simulink model "NHR9410Model96k_2020b"  (R2020b)
settings: Solver=ode45  StartTime=0.0  StopTime=1  FixedStep=0.001  MaxStep=20e-6  RelTol=1e-3
undefined symbols (not defined in the file): Ts
libraries: simulink x85, fl_lib x49, powerlib_meascontrol x27, simulink_extras x24, nesl_utility x13
(part 2 of 4)

== system NHR9410Model96k_2020b/NHR 9410/Chanel-3 ==
  satefy_trip : Inport
  HW Mode Selection : Inport  Port=2
  Ch-3 input [P V I] : Inport  Port=3
  Chanel-3 Control : Subsystem
  Constant : Constant  Value=p_switch
  Constant4 : Constant  Value=0.1
  Current Sensor : fl_lib/Electrical/Electrical Sensors/Current Sensor
  Logical Operator : Logic  AllPortsSameDT=off  OutDataTypeStr=boolean
  Logical Operator1 : Logic  Operator=NOT  AllPortsSameDT=off  OutDataTypeStr=boolean
  NHR 9410 : fl_lib/Electrical/Electrical Sources/Controlled Voltage Source
  PS Constant : fl_lib/Physical Signals/Sources/PS Constant  constant=0
  PS Product1 : fl_lib/Physical Signals/Functions/PS Product
  PS-Simulink Converter1 : nesl_utility/PS-Simulink Converter  PhysicalDomain=network_engine_domain  SubClassName=ps_output  LeftPortType=input  RightPortType=output  PseudoPeriodic=off  Frequencies=[]  Unit=inherit  AffineConversion=off
  PS-Simulink Converter2 : nesl_utility/PS-Simulink Converter  PhysicalDomain=network_engine_domain  SubClassName=ps_output  LeftPortType=input  RightPortType=output  PseudoPeriodic=off  Frequencies=[]  Unit=1  AffineConversion=off
  PS-Simulink Converter4 : nesl_utility/PS-Simulink Converter  PhysicalDomain=network_engine_domain  SubClassName=ps_output  LeftPortType=input  RightPortType=output  PseudoPeriodic=off  Frequencies=[]  Unit=1  AffineConversion=off
  Series Resistor : fl_lib/Electrical/Electrical Elements/Variable Resistor  Rmin=0.0001 Ohm  i_specify=off  i_priority=None  i=0 A  i_nominal_specify=off  i_nominal_unit=A  i_nominal_value=1  v_specify=off  v_priority=None  v=0 V  v_nominal_specify=off  v_nominal_unit=V  v_nominal_value=1
  Simulink-PS Converter : nesl_utility/Simulink-PS Converter  PhysicalDomain=network_engine_domain  SubClassName=ps_input  LeftPortType=input  RightPortType=output  PseudoPeriodic=off  Frequencies=[]  NoiseDistribution=none  NoiseParameters=[]  Unit=1  AffineConversion=off  FilteringAndDerivatives=filter  SimscapeFilterOrder=1  InputFilterTimeConstant=0.001  UdotUserProvided=0
  Switch : Switch  Criteria=u2 > Threshold  ZeroCross=off
  Voltage Sensor1 : fl_lib/Electrical/Electrical Sensors/Voltage Sensor
  + : PMIOPort  Tag=PMCPort  Side=Left
  - : PMIOPort  Tag=PMCPort  Port=2  Side=Left
  Pout : Outport  VectorParamsAs1DForOutWhenUnconnected=off
  Vout : Outport  Port=2  VectorParamsAs1DForOutWhenUnconnected=off
  Iout : Outport  Port=3  VectorParamsAs1DForOutWhenUnconnected=off
  wires:
  PS-Simulink Converter2/1 -> Iout/1, Chanel-3 Control/3(Iout)
  PS-Simulink Converter4/1 -> Vout/1, Chanel-3 Control/2(Vout)
  PS-Simulink Converter1/1 -> Pout/1, Chanel-3 Control/1(Pout)
  HW Mode Selection/1 -> Chanel-3 Control/5(HW mode selection)
  Ch-3 input [P V I]/1 -> Chanel-3 Control/4(Ch-3 input [P V I])
  Constant4/1 -> Switch/3
  Chanel-3 Control/1(Vin) -> Switch/1
  Switch/1 -> Simulink-PS Converter/1
  Logical Operator1/1 -> Logical Operator/2
  satefy_trip/1 -> Logical Operator1/1
  Constant/1 -> Logical Operator/1
  Logical Operator/1 -> Switch/2
  connections:
  Current Sensor/LConn1 -- Series Resistor/RConn1
  PS Constant/RConn1 -- Series Resistor/LConn1
  PS Product1/RConn1 -- PS-Simulink Converter1/LConn1
  Series Resistor/LConn2 -- NHR 9410/LConn1
  Simulink-PS Converter/RConn1 -- NHR 9410/RConn1
  Voltage Sensor1/LConn1 -- +/RConn1 -- Current Sensor/RConn2
  PS-Simulink Converter2/LConn1 -- PS Product1/LConn1 -- Current Sensor/RConn1
  NHR 9410/RConn2 -- -/RConn1 -- Voltage Sensor1/RConn2
  Voltage Sensor1/RConn1 -- PS Product1/LConn2 -- PS-Simulink Converter4/LConn1

== system NHR9410Model96k_2020b/NHR 9410 Safety Settings/Safety Ch-1 ==
  ch-1 out : Inport
  peak_ctrl : Inport  Port=2
  Demux : Demux  Outputs=8
  Logical Operator : Logic  Operator=OR  Inputs=8  AllPortsSameDT=off  OutDataTypeStr=boolean
  Mux : Mux  Inputs=9
  Trip signal generator (max) Sink Current : Subsystem  mask{trip_thres=Imaxsnk1, trip_t=Timaxsnk1}
      mask prompts: trip_thres "Tripping Threshold (max)"; trip_t "Trip Time"
  Trip signal generator (max) Sink Power : Subsystem  mask{trip_thres=Pmaxsnk1, trip_t=Tpmaxsnk1}
      mask prompts: trip_thres "Tripping Threshold (max)"; trip_t "Trip Time"
  Trip signal generator (max) Source Current : Subsystem  mask{trip_thres=Imaxsrc1, trip_t=Timaxsrc1}
      mask prompts: trip_thres "Tripping Threshold (max)"; trip_t "Trip Time"
  Trip signal generator (max) Source Power : Subsystem  mask{trip_thres=Pmaxsrc1, trip_t=Tpmaxsrc1}
      mask prompts: trip_thres "Tripping Threshold (max)"; trip_t "Trip Time"
  Trip signal generator (max) Voltage : Subsystem  mask{trip_thres=Vmax1, trip_t=Tvmax1}
      mask prompts: trip_thres "Tripping Threshold (max)"; trip_t "Trip Time"
  Trip signal generator (min) Voltage : Subsystem  mask{trip_thres=Vmin1, trip_t=Tvmin1}
      mask prompts: trip_thres "Tripping Threshold (max)"; trip_t "Trip Time"
  Trip signal generator (peak) Current : Subsystem  mask{trip_thres=Ipeak1}
      mask prompts: trip_thres "Tripping Threshold (max)"
  Trip signal generator (peak) Voltage : Subsystem  mask{trip_thres=Vpeak1}
      mask prompts: trip_thres "Tripping Threshold (max)"
  ch-1 trip : Outport  VectorParamsAs1DForOutWhenUnconnected=off
  ch-1 trip_all : Outport  Port=2  VectorParamsAs1DForOutWhenUnconnected=off
  wires:
  Demux/1 -> Trip signal generator (min) Voltage/1(signal_in)
  Demux/2 -> Trip signal generator (max) Voltage/1(signal_in)
  Demux/5 -> Trip signal generator (max) Sink Current/1(signal_in)
  Trip signal generator (max) Sink Current/1(signal_trip) -> Mux/6, Logical Operator/5
  Demux/4 -> Trip signal generator (max) Source Current/1(signal_in)
  ch-1 out/1 -> Demux/1
  Trip signal generator (min) Voltage/1(signal_trip) -> Mux/2, Logical Operator/1
  Trip signal generator (max) Source Current/1(signal_trip) -> Mux/5, Logical Operator/4
  Trip signal generator (peak) Voltage/1(signal_trip) -> Mux/4, Logical Operator/3
  Trip signal generator (peak) Current/1(signal_trip) -> Mux/7, Logical Operator/6
  Demux/8 -> Trip signal generator (max) Sink Power/1(signal_in)
  Trip signal generator (max) Voltage/1(signal_trip) -> Mux/3, Logical Operator/2
  Trip signal generator (max) Sink Power/1(signal_trip) -> Mux/9, Logical Operator/8
  Demux/3 -> Trip signal generator (peak) Voltage/1(signal_in)
  Trip signal generator (max) Source Power/1(signal_trip) -> Mux/8, Logical Operator/7
  Demux/7 -> Trip signal generator (max) Source Power/1(signal_in)
  Demux/6 -> Trip signal generator (peak) Current/1(signal_in)
  Logical Operator/1 -> Mux/1, ch-1 trip/1
  peak_ctrl/1 -> Trip signal generator (peak) Voltage/2(peak_ctrl), Trip signal generator (peak) Current/2(peak_ctrl)
  Mux/1 -> ch-1 trip_all/1

== system NHR9410Model96k_2020b/NHR 9410 Safety Settings/Safety Ch-2 ==
  ch-2 out : Inport
  peak_ctrl : Inport  Port=2
  Demux : Demux  Outputs=8
  Logical Operator : Logic  Operator=OR  Inputs=8  AllPortsSameDT=off  OutDataTypeStr=boolean
  Mux : Mux  Inputs=9
  Trip signal generator (max) Sink Current : Subsystem  mask{trip_thres=Imaxsnk2, trip_t=Timaxsnk2}
      mask prompts: trip_thres "Tripping Threshold (max)"; trip_t "Trip Time"
  Trip signal generator (max) Sink Power : Subsystem  mask{trip_thres=Pmaxsnk2, trip_t=Tpmaxsnk2}
      mask prompts: trip_thres "Tripping Threshold (max)"; trip_t "Trip Time"
  Trip signal generator (max) Source Current : Subsystem  mask{trip_thres=Imaxsrc2, trip_t=Timaxsrc2}
      mask prompts: trip_thres "Tripping Threshold (max)"; trip_t "Trip Time"
  Trip signal generator (max) Source Power : Subsystem  mask{trip_thres=Pmaxsrc2, trip_t=Tpmaxsrc2}
      mask prompts: trip_thres "Tripping Threshold (max)"; trip_t "Trip Time"
  Trip signal generator (max) Voltage : Subsystem  mask{trip_thres=Vmax2, trip_t=Tvmax2}
      mask prompts: trip_thres "Tripping Threshold (max)"; trip_t "Trip Time"
  Trip signal generator (min) Voltage : Subsystem  mask{trip_thres=Vmin2, trip_t=Tvmin2}
      mask prompts: trip_thres "Tripping Threshold (max)"; trip_t "Trip Time"
  Trip signal generator (peak) Current : Subsystem  mask{trip_thres=Ipeak2}
      mask prompts: trip_thres "Tripping Threshold (max)"
  Trip signal generator (peak) Voltage : Subsystem  mask{trip_thres=Vpeak2}
      mask prompts: trip_thres "Tripping Threshold (max)"
  ch-2 trip : Outport  VectorParamsAs1DForOutWhenUnconnected=off
  ch-2 trip_all : Outport  Port=2  VectorParamsAs1DForOutWhenUnconnected=off
  wires:
  Logical Operator/1 -> Mux/1, ch-2 trip/1
  Demux/6 -> Trip signal generator (peak) Current/1(signal_in)
  Demux/7 -> Trip signal generator (max) Source Power/1(signal_in)
  Trip signal generator (max) Source Power/1(signal_trip) -> Mux/8, Logical Operator/7
  Demux/3 -> Trip signal generator (peak) Voltage/1(signal_in)
  Trip signal generator (max) Sink Power/1(signal_trip) -> Mux/9, Logical Operator/8
  Trip signal generator (max) Voltage/1(signal_trip) -> Mux/3, Logical Operator/2
  Demux/8 -> Trip signal generator (max) Sink Power/1(signal_in)
  Trip signal generator (peak) Current/1(signal_trip) -> Mux/7, Logical Operator/6
  Trip signal generator (peak) Voltage/1(signal_trip) -> Mux/4, Logical Operator/3
  Trip signal generator (max) Source Current/1(signal_trip) -> Mux/5, Logical Operator/4
  Trip signal generator (min) Voltage/1(signal_trip) -> Mux/2, Logical Operator/1
  ch-2 out/1 -> Demux/1
  Demux/4 -> Trip signal generator (max) Source Current/1(signal_in)
  Demux/5 -> Trip signal generator (max) Sink Current/1(signal_in)
  Demux/2 -> Trip signal generator (max) Voltage/1(signal_in)
  Demux/1 -> Trip signal generator (min) Voltage/1(signal_in)
  peak_ctrl/1 -> Trip signal generator (peak) Voltage/2(peak_ctrl), Trip signal generator (peak) Current/2(peak_ctrl)
  Mux/1 -> ch-2 trip_all/1
  Trip signal generator (max) Sink Current/1(signal_trip) -> Mux/6, Logical Operator/5

== system NHR9410Model96k_2020b/NHR 9410 Safety Settings/Safety Ch-3 ==
  ch-3 out : Inport
  peak_ctrl : Inport  Port=2
  Demux : Demux  Outputs=8
  Logical Operator : Logic  Operator=OR  Inputs=8  AllPortsSameDT=off  OutDataTypeStr=boolean
  Mux : Mux  Inputs=9
  Trip signal generator (max) Sink Current : Subsystem  mask{trip_thres=Imaxsnk3, trip_t=Timaxsnk3}
      mask prompts: trip_thres "Tripping Threshold (max)"; trip_t "Trip Time"
  Trip signal generator (max) Sink Power : Subsystem  mask{trip_thres=Pmaxsnk3, trip_t=Tpmaxsnk3}
      mask prompts: trip_thres "Tripping Threshold (max)"; trip_t "Trip Time"
  Trip signal generator (max) Source Current : Subsystem  mask{trip_thres=Imaxsrc3, trip_t=Timaxsrc3}
      mask prompts: trip_thres "Tripping Threshold (max)"; trip_t "Trip Time"
  Trip signal generator (max) Source Power : Subsystem  mask{trip_thres=Pmaxsrc3, trip_t=Tpmaxsrc3}
      mask prompts: trip_thres "Tripping Threshold (max)"; trip_t "Trip Time"
  Trip signal generator (max) Voltage : Subsystem  mask{trip_thres=Vmax3, trip_t=Tvmax3}
      mask prompts: trip_thres "Tripping Threshold (max)"; trip_t "Trip Time"
  Trip signal generator (min) Voltage : Subsystem  mask{trip_thres=Vmin3, trip_t=Tvmin3}
      mask prompts: trip_thres "Tripping Threshold (max)"; trip_t "Trip Time"
  Trip signal generator (peak) Current : Subsystem  mask{trip_thres=Ipeak3}
      mask prompts: trip_thres "Tripping Threshold (max)"
  Trip signal generator (peak) Voltage : Subsystem  mask{trip_thres=Vpeak3}
      mask prompts: trip_thres "Tripping Threshold (max)"
  ch-3 trip : Outport  VectorParamsAs1DForOutWhenUnconnected=off
  ch-3 trip_all : Outport  Port=2  VectorParamsAs1DForOutWhenUnconnected=off
  wires:
  Demux/1 -> Trip signal generator (min) Voltage/1(signal_in)
  Demux/2 -> Trip signal generator (max) Voltage/1(signal_in)
  Demux/5 -> Trip signal generator (max) Sink Current/1(signal_in)
  Trip signal generator (max) Sink Current/1(signal_trip) -> Mux/6, Logical Operator/5
  Demux/4 -> Trip signal generator (max) Source Current/1(signal_in)
  ch-3 out/1 -> Demux/1
  Trip signal generator (min) Voltage/1(signal_trip) -> Mux/2, Logical Operator/1
  Trip signal generator (max) Source Current/1(signal_trip) -> Mux/5, Logical Operator/4
  Trip signal generator (peak) Voltage/1(signal_trip) -> Mux/4, Logical Operator/3
  Trip signal generator (peak) Current/1(signal_trip) -> Mux/7, Logical Operator/6
  Demux/8 -> Trip signal generator (max) Sink Power/1(signal_in)
  Trip signal generator (max) Voltage/1(signal_trip) -> Mux/3, Logical Operator/2
  Trip signal generator (max) Sink Power/1(signal_trip) -> Mux/9, Logical Operator/8
  Demux/3 -> Trip signal generator (peak) Voltage/1(signal_in)
  Trip signal generator (max) Source Power/1(signal_trip) -> Mux/8, Logical Operator/7
  Demux/7 -> Trip signal generator (max) Source Power/1(signal_in)
  Demux/6 -> Trip signal generator (peak) Current/1(signal_in)
  Logical Operator/1 -> Mux/1, ch-3 trip/1
  peak_ctrl/1 -> Trip signal generator (peak) Current/2(peak_ctrl), Trip signal generator (peak) Voltage/2(peak_ctrl)
  Mux/1 -> ch-3 trip_all/1

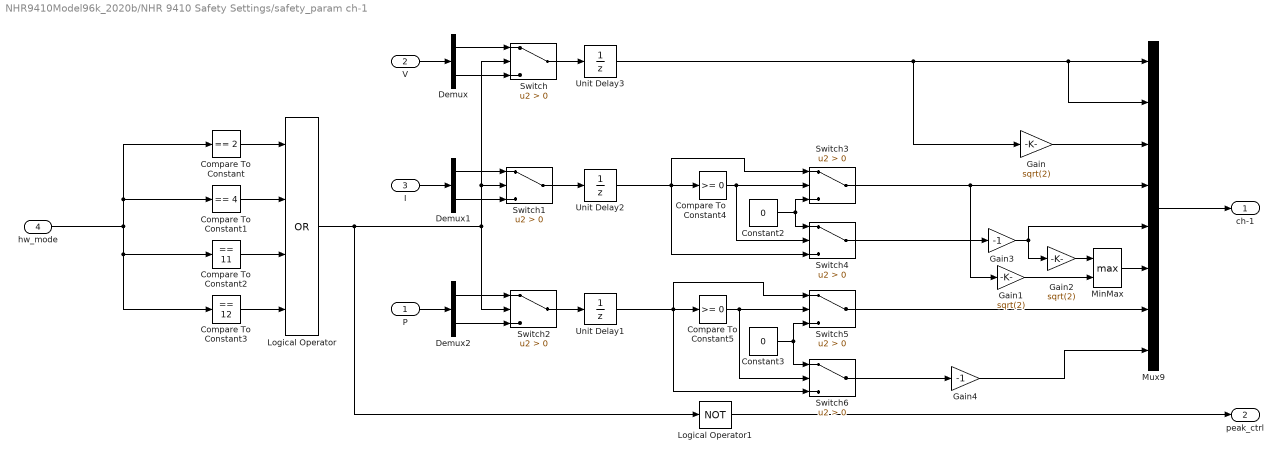
== system NHR9410Model96k_2020b/NHR 9410 Safety Settings/safety_param ch-1 ==
  P : Inport
  V : Inport  Port=2
  I : Inport  Port=3
  hw_mode : Inport  Port=4
  Compare To Constant : simulink/Logic and Bit Operations/Compare To Constant  relop===  const=2  OutDataTypeStr=boolean
  Compare To Constant1 : simulink/Logic and Bit Operations/Compare To Constant  relop===  const=4  OutDataTypeStr=boolean
  Compare To Constant2 : simulink/Logic and Bit Operations/Compare To Constant  relop===  const=11  OutDataTypeStr=boolean
  Compare To Constant3 : simulink/Logic and Bit Operations/Compare To Constant  relop===  const=12  OutDataTypeStr=boolean
  Compare To Constant4 : simulink/Logic and Bit Operations/Compare To Constant  relop=>=  const=0  OutDataTypeStr=boolean
  Compare To Constant5 : simulink/Logic and Bit Operations/Compare To Constant  relop=>=  const=0  OutDataTypeStr=boolean
  Constant2 : Constant  Value=0
  Constant3 : Constant  Value=0
  Demux : Demux  Outputs=2
  Demux1 : Demux  Outputs=2
  Demux2 : Demux  Outputs=2
  Gain : Gain  Gain=sqrt(2)
  Gain1 : Gain  Gain=sqrt(2)
  Gain2 : Gain  Gain=sqrt(2)
  Gain3 : Gain  Gain=-1
  Gain4 : Gain  Gain=-1
  Logical Operator : Logic  Operator=OR  Inputs=4  AllPortsSameDT=off  OutDataTypeStr=boolean
  Logical Operator1 : Logic  Operator=NOT  Inputs=4  AllPortsSameDT=off  OutDataTypeStr=boolean
  MinMax : MinMax  Function=max  Inputs=2
  Mux9 : Mux  Inputs=8
  Switch{,1..6} (7 alike) : Switch  Criteria=u2 > Threshold
  Unit Delay1 : UnitDelay  SampleTime=-1  HasFrameUpgradeWarning=on
  Unit Delay2 : UnitDelay  SampleTime=-1  HasFrameUpgradeWarning=on
  Unit Delay3 : UnitDelay  SampleTime=-1  HasFrameUpgradeWarning=on
  ch-1 : Outport  VectorParamsAs1DForOutWhenUnconnected=off
  peak_ctrl : Outport  Port=2  VectorParamsAs1DForOutWhenUnconnected=off
  wires:
  Mux9/1 -> ch-1/1
  Switch4/1 -> Gain3/1
  V/1 -> Demux/1
  I/1 -> Demux1/1
  P/1 -> Demux2/1
  Demux1/2 -> Switch1/3
  hw_mode/1 -> Compare To Constant3/1, Compare To Constant2/1, Compare To Constant1/1, Compare To Constant/1
  Demux2/2 -> Switch2/3
  Switch2/1 -> Unit Delay1/1
  Gain/1 -> Mux9/3
  Compare To Constant/1 -> Logical Operator/1
  Compare To Constant1/1 -> Logical Operator/2
  Compare To Constant2/1 -> Logical Operator/3
  Compare To Constant3/1 -> Logical Operator/4
  Demux/1 -> Switch/1
  Demux/2 -> Switch/3
  Switch/1 -> Unit Delay3/1
  Demux1/1 -> Switch1/1
  Demux2/1 -> Switch2/1
  Logical Operator/1 -> Logical Operator1/1, Switch/2, Switch1/2, Switch2/2
  MinMax/1 -> Mux9/6
  Gain1/1 -> MinMax/2
  Gain2/1 -> MinMax/1
  Gain4/1 -> Mux9/8
  Logical Operator1/1 -> peak_ctrl/1
  Compare To Constant4/1 -> Switch4/2, Switch3/2
  Constant2/1 -> Switch4/1, Switch3/3
  Switch1/1 -> Unit Delay2/1
  Gain3/1 -> Gain2/1, Mux9/5
  Compare To Constant5/1 -> Switch6/2, Switch5/2
  Constant3/1 -> Switch6/1, Switch5/3
  Switch5/1 -> Mux9/7
  Switch6/1 -> Gain4/1
  Unit Delay1/1 -> Switch6/3, Compare To Constant5/1, Switch5/1
  Unit Delay2/1 -> Switch4/3, Switch3/1, Compare To Constant4/1
  Unit Delay3/1 -> Mux9/2, Mux9/1, Gain/1
  Switch3/1 -> Gain1/1, Mux9/4

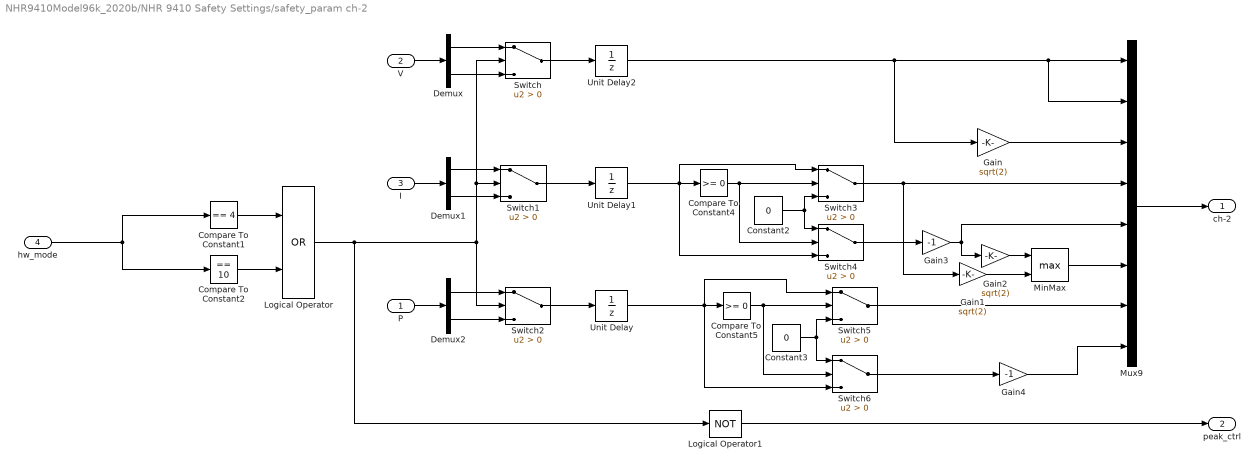
== system NHR9410Model96k_2020b/NHR 9410 Safety Settings/safety_param ch-2 ==
  P : Inport
  V : Inport  Port=2
  I : Inport  Port=3
  hw_mode : Inport  Port=4
  Compare To Constant1 : simulink/Logic and Bit Operations/Compare To Constant  relop===  const=4  OutDataTypeStr=boolean
  Compare To Constant2 : simulink/Logic and Bit Operations/Compare To Constant  relop===  const=10  OutDataTypeStr=boolean
  Compare To Constant4 : simulink/Logic and Bit Operations/Compare To Constant  relop=>=  const=0  OutDataTypeStr=boolean
  Compare To Constant5 : simulink/Logic and Bit Operations/Compare To Constant  relop=>=  const=0  OutDataTypeStr=boolean
  Constant2 : Constant  Value=0
  Constant3 : Constant  Value=0
  Demux : Demux  Outputs=2
  Demux1 : Demux  Outputs=2
  Demux2 : Demux  Outputs=2
  Gain : Gain  Gain=sqrt(2)
  Gain1 : Gain  Gain=sqrt(2)
  Gain2 : Gain  Gain=sqrt(2)
  Gain3 : Gain  Gain=-1
  Gain4 : Gain  Gain=-1
  Logical Operator : Logic  Operator=OR  AllPortsSameDT=off  OutDataTypeStr=boolean
  Logical Operator1 : Logic  Operator=NOT  Inputs=4  AllPortsSameDT=off  OutDataTypeStr=boolean
  MinMax : MinMax  Function=max  Inputs=2
  Mux9 : Mux  Inputs=8
  Switch{,1..6} (7 alike) : Switch  Criteria=u2 > Threshold
  Unit Delay : UnitDelay  SampleTime=-1  HasFrameUpgradeWarning=on
  Unit Delay1 : UnitDelay  SampleTime=-1  HasFrameUpgradeWarning=on
  Unit Delay2 : UnitDelay  SampleTime=-1  HasFrameUpgradeWarning=on
  ch-2 : Outport  VectorParamsAs1DForOutWhenUnconnected=off
  peak_ctrl : Outport  Port=2  VectorParamsAs1DForOutWhenUnconnected=off
  wires:
  Gain2/1 -> MinMax/1
  Gain1/1 -> MinMax/2
  MinMax/1 -> Mux9/6
  Demux2/1 -> Switch2/1
  Demux1/1 -> Switch1/1
  Switch/1 -> Unit Delay2/1
  Demux/2 -> Switch/3
  Demux/1 -> Switch/1
  Compare To Constant2/1 -> Logical Operator/2
  Compare To Constant1/1 -> Logical Operator/1
  Gain/1 -> Mux9/3
  Demux2/2 -> Switch2/3
  hw_mode/1 -> Compare To Constant1/1, Compare To Constant2/1
  Demux1/2 -> Switch1/3
  P/1 -> Demux2/1
  I/1 -> Demux1/1
  V/1 -> Demux/1
  Mux9/1 -> ch-2/1
  Logical Operator/1 -> Logical Operator1/1, Switch2/2, Switch1/2, Switch/2
  Logical Operator1/1 -> peak_ctrl/1
  Switch2/1 -> Unit Delay/1
  Switch5/1 -> Mux9/7
  Constant3/1 -> Switch6/1, Switch5/3
  Compare To Constant5/1 -> Switch6/2, Switch5/2
  Switch6/1 -> Gain4/1
  Gain4/1 -> Mux9/8
  Switch1/1 -> Unit Delay1/1
  Constant2/1 -> Switch4/1, Switch3/3
  Compare To Constant4/1 -> Switch3/2, Switch4/2
  Switch3/1 -> Gain1/1, Mux9/4
  Switch4/1 -> Gain3/1
  Gain3/1 -> Gain2/1, Mux9/5
  Unit Delay/1 -> Switch6/3, Switch5/1, Compare To Constant5/1
  Unit Delay1/1 -> Compare To Constant4/1, Switch4/3, Switch3/1
  Unit Delay2/1 -> Gain/1, Mux9/1, Mux9/2

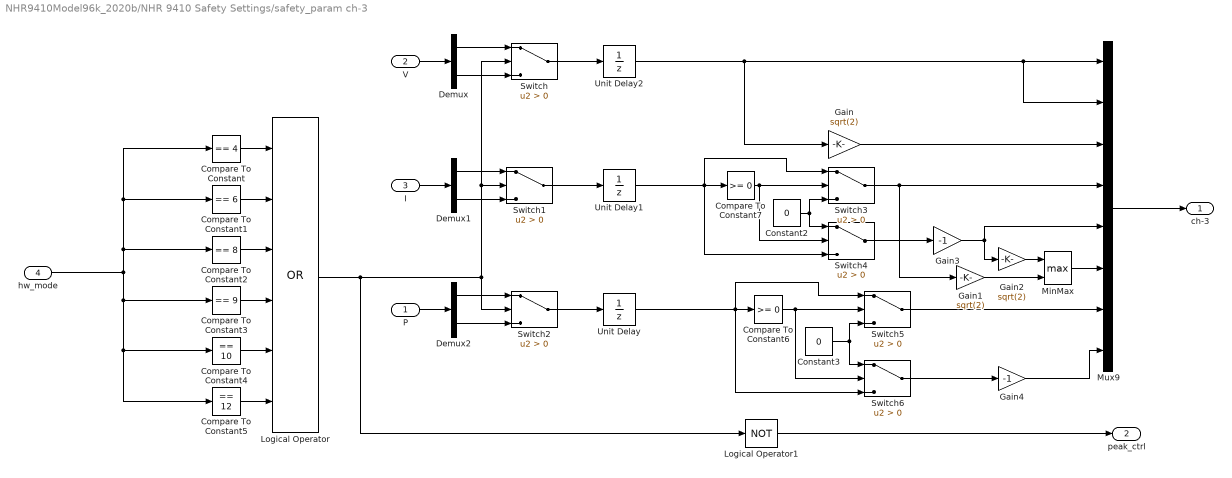
== system NHR9410Model96k_2020b/NHR 9410 Safety Settings/safety_param ch-3 ==
  P : Inport
  V : Inport  Port=2
  I : Inport  Port=3
  hw_mode : Inport  Port=4
  Compare To Constant : simulink/Logic and Bit Operations/Compare To Constant  relop===  const=4  OutDataTypeStr=boolean
  Compare To Constant1 : simulink/Logic and Bit Operations/Compare To Constant  relop===  const=6  OutDataTypeStr=boolean
  Compare To Constant2 : simulink/Logic and Bit Operations/Compare To Constant  relop===  const=8  OutDataTypeStr=boolean
  Compare To Constant3 : simulink/Logic and Bit Operations/Compare To Constant  relop===  const=9  OutDataTypeStr=boolean
  Compare To Constant4 : simulink/Logic and Bit Operations/Compare To Constant  relop===  const=10  OutDataTypeStr=boolean
  Compare To Constant5 : simulink/Logic and Bit Operations/Compare To Constant  relop===  const=12  OutDataTypeStr=boolean
  Compare To Constant6 : simulink/Logic and Bit Operations/Compare To Constant  relop=>=  const=0  OutDataTypeStr=boolean
  Compare To Constant7 : simulink/Logic and Bit Operations/Compare To Constant  relop=>=  const=0  OutDataTypeStr=boolean
  Constant2 : Constant  Value=0
  Constant3 : Constant  Value=0
  Demux : Demux  Outputs=2
  Demux1 : Demux  Outputs=2
  Demux2 : Demux  Outputs=2
  Gain : Gain  Gain=sqrt(2)
  Gain1 : Gain  Gain=sqrt(2)
  Gain2 : Gain  Gain=sqrt(2)
  Gain3 : Gain  Gain=-1
  Gain4 : Gain  Gain=-1
  Logical Operator : Logic  Operator=OR  Inputs=6  AllPortsSameDT=off  OutDataTypeStr=boolean
  Logical Operator1 : Logic  Operator=NOT  Inputs=4  AllPortsSameDT=off  OutDataTypeStr=boolean
  MinMax : MinMax  Function=max  Inputs=2
  Mux9 : Mux  Inputs=8
  Switch{,1..6} (7 alike) : Switch  Criteria=u2 > Threshold
  Unit Delay : UnitDelay  SampleTime=-1  HasFrameUpgradeWarning=on
  Unit Delay1 : UnitDelay  SampleTime=-1  HasFrameUpgradeWarning=on
  Unit Delay2 : UnitDelay  SampleTime=-1  HasFrameUpgradeWarning=on
  ch-3 : Outport  VectorParamsAs1DForOutWhenUnconnected=off
  peak_ctrl : Outport  Port=2  VectorParamsAs1DForOutWhenUnconnected=off
  wires:
  Mux9/1 -> ch-3/1
  V/1 -> Demux/1
  I/1 -> Demux1/1
  P/1 -> Demux2/1
  Demux1/2 -> Switch1/3
  hw_mode/1 -> Compare To Constant1/1, Compare To Constant/1, Compare To Constant2/1, Compare To Constant5/1, Compare To Constant4/1, Compare To Constant3/1
  Demux2/2 -> Switch2/3
  Gain/1 -> Mux9/3
  Demux/1 -> Switch/1
  Demux/2 -> Switch/3
  Switch/1 -> Unit Delay2/1
  Demux1/1 -> Switch1/1
  Demux2/1 -> Switch2/1
  MinMax/1 -> Mux9/6
  Gain1/1 -> MinMax/2
  Gain2/1 -> MinMax/1
  Compare To Constant/1 -> Logical Operator/1
  Compare To Constant1/1 -> Logical Operator/2
  Compare To Constant2/1 -> Logical Operator/3
  Compare To Constant3/1 -> Logical Operator/4
  Compare To Constant4/1 -> Logical Operator/5
  Compare To Constant5/1 -> Logical Operator/6
  Logical Operator/1 -> Logical Operator1/1, Switch/2, Switch1/2, Switch2/2
  Logical Operator1/1 -> peak_ctrl/1
  Switch2/1 -> Unit Delay/1
  Switch5/1 -> Mux9/7
  Constant3/1 -> Switch6/1, Switch5/3
  Compare To Constant6/1 -> Switch6/2, Switch5/2
  Switch6/1 -> Gain4/1
  Gain4/1 -> Mux9/8
  Constant2/1 -> Switch4/1, Switch3/3
  Switch1/1 -> Unit Delay1/1
  Compare To Constant7/1 -> Switch4/2, Switch3/2
  Switch4/1 -> Gain3/1
  Gain3/1 -> Mux9/5, Gain2/1
  Switch3/1 -> Mux9/4, Gain1/1
  Unit Delay/1 -> Compare To Constant6/1, Switch6/3, Switch5/1
  Unit Delay1/1 -> Compare To Constant7/1, Switch3/1, Switch4/3
  Unit Delay2/1 -> Mux9/2, Mux9/1, Gain/1

== system NHR9410Model96k_2020b/NHR 9410-96k Input Panel/Default: 0 inputs ==
  Mux3 : Mux  Inputs=3
  ch-1 : Constant  Value=[0,0,0]
  ch-2 : Constant  Value=[0,0,0]
  ch-3 : Constant  Value=[0,0,0]
  ch [1 2 3] : Outport  VectorParamsAs1DForOutWhenUnconnected=off
  wires:
  Mux3/1 -> ch [1 2 3]/1
  ch-1/1 -> Mux3/1
  ch-2/1 -> Mux3/2
  ch-3/1 -> Mux3/3

== system NHR9410Model96k_2020b/NHR 9410-96k Input Panel/mode0 ==
  Angle-1 : Constant  Value=0
  Angle-2 : Constant  Value=240
  Angle-3 : Constant  Value=120
  Frequency-1 : Constant  Value=md0f1
  Gain : Gain  Gain=1000
  Mux{,1..3} (4 alike) : Mux  Inputs=3
  Mux4 : Mux  Inputs=6
  ch-1 current : Constant  Value=md0Irms1
  ch-1 power : Constant  Value=md0Pm1/3
  ch-1 voltage : Constant  Value=md0Vrms1
  ch [1 2 3] : Outport  VectorParamsAs1DForOutWhenUnconnected=off
  F [Angles-1,2,3] : Outport  Port=2  VectorParamsAs1DForOutWhenUnconnected=off
  wires:
  ch-1 voltage/1 -> Mux2/2, Mux1/2, Mux/2
  Mux4/1 -> F [Angles-1,2,3]/1
  Mux3/1 -> ch [1 2 3]/1
  ch-1 current/1 -> Mux1/3, Mux2/3, Mux/3
  Mux1/1 -> Mux3/2
  Mux/1 -> Mux3/1
  Mux2/1 -> Mux3/3
  Gain/1 -> Mux2/1, Mux1/1, Mux/1
  ch-1 power/1 -> Gain/1
  Angle-3/1 -> Mux4/6
  Angle-2/1 -> Mux4/5
  Angle-1/1 -> Mux4/4
  Frequency-1/1 -> Mux4/3, Mux4/2, Mux4/1

== system NHR9410Model96k_2020b/NHR 9410-96k Input Panel/mode1 ==
  Angle-1 : Constant  Value=md1ph
  Angle-2 : Constant  Value=0
  Angle-3 : Constant  Value=0
  Frequency-1 : Constant  Value=md1f
  Frequency-2 : Constant  Value=0
  Frequency-3 : Constant  Value=0
  Gain : Gain  Gain=1000
  Gain1 : Gain  Gain=1000
  Gain2 : Gain  Gain=1000
  Mux{,1..3} (4 alike) : Mux  Inputs=3
  Mux5 : Mux  Inputs=6
  ch-1 current : Constant  Value=md1Irms
  ch-1 power : Constant  Value=md1Pm
  ch-1 voltage : Constant  Value=md1Vrms
  ch-2 current : Constant  Value=0
  ch-2 power : Constant  Value=0
  ch-2 voltage : Constant  Value=0
  ch-3 current : Constant  Value=0
  ch-3 power : Constant  Value=0
  ch-3 voltage : Constant  Value=0
  ch [1 2 3] : Outport  VectorParamsAs1DForOutWhenUnconnected=off
  F [Angles-1,2,3] : Outport  Port=2  VectorParamsAs1DForOutWhenUnconnected=off
  wires:
  Gain2/1 -> Mux2/1
  Gain1/1 -> Mux1/1
  ch-1 power/1 -> Gain/1
  Gain/1 -> Mux/1
  Mux2/1 -> Mux3/3
  Mux/1 -> Mux3/1
  Mux1/1 -> Mux3/2
  ch-3 power/1 -> Gain2/1
  ch-3 voltage/1 -> Mux2/2
  ch-3 current/1 -> Mux2/3
  ch-2 current/1 -> Mux1/3
  ch-2 voltage/1 -> Mux1/2
  ch-2 power/1 -> Gain1/1
  ch-1 current/1 -> Mux/3
  Mux3/1 -> ch [1 2 3]/1
  ch-1 voltage/1 -> Mux/2
  Angle-1/1 -> Mux5/4
  Frequency-2/1 -> Mux5/2
  Frequency-3/1 -> Mux5/3
  Angle-2/1 -> Mux5/5
  Angle-3/1 -> Mux5/6
  Frequency-1/1 -> Mux5/1
  Mux5/1 -> F [Angles-1,2,3]/1

== system NHR9410Model96k_2020b/NHR 9410-96k Input Panel/mode10 ==
  Angle-1 : Constant  Value=md10ph1
  Angle-2 : Constant  Value=0
  Angle-3 : Constant  Value=0
  Frequency-1 : Constant  Value=md10f1
  Frequency-2 : Constant  Value=0
  Frequency-3 : Constant  Value=0
  Gain : Gain  Gain=1000
  Gain1 : Gain  Gain=1000
  Gain2 : Gain  Gain=1000
  Mux{,1..3} (4 alike) : Mux  Inputs=3
  Mux5 : Mux  Inputs=6
  ch-1 current : Constant  Value=md10Irms1
  ch-1 power : Constant  Value=md10Pm1
  ch-1 voltage : Constant  Value=md10Vrms1
  ch-2 current : Constant  Value=md10Im2
  ch-2 power : Constant  Value=md10Pm2
  ch-2 voltage : Constant  Value=md10Vm2
  ch-3 current : Constant  Value=md10Im3
  ch-3 power : Constant  Value=md10Pm3
  ch-3 voltage : Constant  Value=md10Vm3
  ch [1 2 3] : Outport  VectorParamsAs1DForOutWhenUnconnected=off
  F [Angles-1,2,3] : Outport  Port=2  VectorParamsAs1DForOutWhenUnconnected=off
  wires:
  ch-1 voltage/1 -> Mux/2
  Mux3/1 -> ch [1 2 3]/1
  ch-1 current/1 -> Mux/3
  ch-2 power/1 -> Gain1/1
  ch-2 voltage/1 -> Mux1/2
  ch-2 current/1 -> Mux1/3
  ch-3 current/1 -> Mux2/3
  ch-3 voltage/1 -> Mux2/2
  ch-3 power/1 -> Gain2/1
  Mux1/1 -> Mux3/2
  Mux/1 -> Mux3/1
  Mux2/1 -> Mux3/3
  Gain/1 -> Mux/1
  ch-1 power/1 -> Gain/1
  Gain1/1 -> Mux1/1
  Gain2/1 -> Mux2/1
  Angle-1/1 -> Mux5/4
  Frequency-2/1 -> Mux5/2
  Frequency-3/1 -> Mux5/3
  Angle-2/1 -> Mux5/5
  Angle-3/1 -> Mux5/6
  Frequency-1/1 -> Mux5/1
  Mux5/1 -> F [Angles-1,2,3]/1

== system NHR9410Model96k_2020b/NHR 9410-96k Input Panel/mode11 ==
  Angle-1 : Constant  Value=0
  Angle-2 : Constant  Value=0
  Angle-3 : Constant  Value=md11ph2
  Frequency-1 : Constant  Value=0
  Frequency-2 : Constant  Value=0
  Frequency-3 : Constant  Value=md11f2
  Gain : Gain  Gain=1000
  Gain1 : Gain  Gain=1000
  Gain2 : Gain  Gain=1000
  Mux{,1..3} (4 alike) : Mux  Inputs=3
  Mux5 : Mux  Inputs=6
  ch-1 current : Constant  Value=md11Im1
  ch-1 power : Constant  Value=md11Pm1
  ch-1 voltage : Constant  Value=md11Vm1
  ch-2 current : Constant  Value=0
  ch-2 power : Constant  Value=0
  ch-2 voltage : Constant  Value=0
  ch-3 current : Constant  Value=md11Irms2
  ch-3 power : Constant  Value=md11Pm2
  ch-3 voltage : Constant  Value=md11Vrms2
  ch [1 2 3] : Outport  VectorParamsAs1DForOutWhenUnconnected=off
  F [Angles-1,2,3] : Outport  Port=2  VectorParamsAs1DForOutWhenUnconnected=off
  wires:
  ch-1 voltage/1 -> Mux/2
  Mux3/1 -> ch [1 2 3]/1
  ch-1 current/1 -> Mux/3
  ch-2 power/1 -> Gain1/1
  ch-2 voltage/1 -> Mux1/2
  ch-2 current/1 -> Mux1/3
  ch-3 current/1 -> Mux2/3
  ch-3 voltage/1 -> Mux2/2
  ch-3 power/1 -> Gain2/1
  Mux1/1 -> Mux3/2
  Mux/1 -> Mux3/1
  Mux2/1 -> Mux3/3
  Gain/1 -> Mux/1
  ch-1 power/1 -> Gain/1
  Gain1/1 -> Mux1/1
  Gain2/1 -> Mux2/1
  Angle-1/1 -> Mux5/4
  Frequency-2/1 -> Mux5/2
  Frequency-3/1 -> Mux5/3
  Angle-2/1 -> Mux5/5
  Angle-3/1 -> Mux5/6
  Frequency-1/1 -> Mux5/1
  Mux5/1 -> F [Angles-1,2,3]/1

== system NHR9410Model96k_2020b/NHR 9410-96k Input Panel/mode12 ==
  Gain : Gain  Gain=1000
  Gain1 : Gain  Gain=1000
  Gain2 : Gain  Gain=1000
  Mux{,1..3} (4 alike) : Mux  Inputs=3
  ch-1 current : Constant  Value=md12Im1
  ch-1 power : Constant  Value=md12Pm1
  ch-1 voltage : Constant  Value=md12Vm1
  ch-2 current : Constant  Value=0
  ch-2 power : Constant  Value=0
  ch-2 voltage : Constant  Value=0
  ch-3 current : Constant  Value=md12Im2
  ch-3 power : Constant  Value=md12Pm2
  ch-3 voltage : Constant  Value=md12Vm2
  ch [1 2 3] : Outport  VectorParamsAs1DForOutWhenUnconnected=off
  wires:
  Gain2/1 -> Mux2/1
  Gain1/1 -> Mux1/1
  ch-1 power/1 -> Gain/1
  Gain/1 -> Mux/1
  Mux2/1 -> Mux3/3
  Mux/1 -> Mux3/1
  Mux1/1 -> Mux3/2
  ch-3 power/1 -> Gain2/1
  ch-3 voltage/1 -> Mux2/2
  ch-3 current/1 -> Mux2/3
  ch-2 current/1 -> Mux1/3
  ch-2 voltage/1 -> Mux1/2
  ch-2 power/1 -> Gain1/1
  ch-1 current/1 -> Mux/3
  ch-1 voltage/1 -> Mux/2
  Mux3/1 -> ch [1 2 3]/1

== system NHR9410Model96k_2020b/NHR 9410-96k Input Panel/mode2 ==
  Gain : Gain  Gain=1000
  Gain1 : Gain  Gain=1000
  Gain2 : Gain  Gain=1000
  Mux{,1..3} (4 alike) : Mux  Inputs=3
  ch-1 Current : Constant  Value=md2Im
  ch-1 Voltage : Constant  Value=md2Vm
  ch-1 power : Constant  Value=md2Pm
  ch-2 Current : Constant  Value=0
  ch-2 Voltage : Constant  Value=0
  ch-2 power : Constant  Value=0
  ch-3 Current : Constant  Value=0
  ch-3 Voltage : Constant  Value=0
  ch-3 power : Constant  Value=0
  ch [1 2 3] : Outport  VectorParamsAs1DForOutWhenUnconnected=off
  wires:
  Mux3/1 -> ch [1 2 3]/1
  ch-1 Voltage/1 -> Mux/2
  ch-1 Current/1 -> Mux/3
  ch-2 power/1 -> Gain1/1
  ch-2 Voltage/1 -> Mux1/2
  ch-2 Current/1 -> Mux1/3
  ch-3 Current/1 -> Mux2/3
  ch-3 Voltage/1 -> Mux2/2
  ch-3 power/1 -> Gain2/1
  Mux1/1 -> Mux3/2
  Mux/1 -> Mux3/1
  Mux2/1 -> Mux3/3
  Gain/1 -> Mux/1
  ch-1 power/1 -> Gain/1
  Gain1/1 -> Mux1/1
  Gain2/1 -> Mux2/1

== system NHR9410Model96k_2020b/NHR 9410-96k Input Panel/mode3 ==
  Angle-1 : Constant  Value=md3ph1
  Angle-2 : Constant  Value=md3ph2
  Angle-3 : Constant  Value=md3ph3
  Frequency-1 : Constant  Value=md3f1
  Frequency-2 : Constant  Value=md3f2
  Frequency-3 : Constant  Value=md3f3
  Gain : Gain  Gain=1000
  Gain1 : Gain  Gain=1000
  Gain2 : Gain  Gain=1000
  Mux{,1..3} (4 alike) : Mux  Inputs=3
  Mux5 : Mux  Inputs=6
  ch-1 current : Constant  Value=md3Irms1
  ch-1 power : Constant  Value=md3Pm1
  ch-1 voltage : Constant  Value=md3Vrms1
  ch-2 current : Constant  Value=md3Irms2
  ch-2 power : Constant  Value=md3Pm2
  ch-2 voltage : Constant  Value=md3Vrms2
  ch-3 current : Constant  Value=md3Irms3
  ch-3 power : Constant  Value=md3Pm3
  ch-3 voltage : Constant  Value=md3Vrms3
  ch [1 2 3] : Outport  VectorParamsAs1DForOutWhenUnconnected=off
  F [Angles-1,2,3] : Outport  Port=2  VectorParamsAs1DForOutWhenUnconnected=off
  wires:
  Gain2/1 -> Mux2/1
  Gain1/1 -> Mux1/1
  ch-1 power/1 -> Gain/1
  Gain/1 -> Mux/1
  Mux2/1 -> Mux3/3
  Mux/1 -> Mux3/1
  Mux1/1 -> Mux3/2
  ch-3 power/1 -> Gain2/1
  ch-3 voltage/1 -> Mux2/2
  ch-3 current/1 -> Mux2/3
  ch-2 current/1 -> Mux1/3
  ch-2 voltage/1 -> Mux1/2
  ch-2 power/1 -> Gain1/1
  ch-1 current/1 -> Mux/3
  Mux3/1 -> ch [1 2 3]/1
  ch-1 voltage/1 -> Mux/2
  Angle-1/1 -> Mux5/4
  Frequency-2/1 -> Mux5/2
  Frequency-3/1 -> Mux5/3
  Angle-3/1 -> Mux5/6
  Frequency-1/1 -> Mux5/1
  Angle-2/1 -> Mux5/5
  Mux5/1 -> F [Angles-1,2,3]/1

== system NHR9410Model96k_2020b/NHR 9410-96k Input Panel/mode4 ==
  Gain : Gain  Gain=1000
  Gain1 : Gain  Gain=1000
  Gain2 : Gain  Gain=1000
  Mux{,1..3} (4 alike) : Mux  Inputs=3
  ch-1 current : Constant  Value=md4Im1
  ch-1 power : Constant  Value=md4Pm1
  ch-1 voltage : Constant  Value=md4Vm1
  ch-2 current : Constant  Value=md4Im2
  ch-2 power : Constant  Value=md4Pm2
  ch-2 voltage : Constant  Value=md4Vm2
  ch-3 current : Constant  Value=md4Im2
  ch-3 power : Constant  Value=md4Pm3
  ch-3 voltage : Constant  Value=md4Vm2
  ch [1 2 3] : Outport  VectorParamsAs1DForOutWhenUnconnected=off
  wires:
  Gain2/1 -> Mux2/1
  Gain1/1 -> Mux1/1
  ch-1 power/1 -> Gain/1
  Gain/1 -> Mux/1
  Mux2/1 -> Mux3/3
  Mux/1 -> Mux3/1
  Mux1/1 -> Mux3/2
  ch-3 power/1 -> Gain2/1
  ch-3 voltage/1 -> Mux2/2
  ch-3 current/1 -> Mux2/3
  ch-2 current/1 -> Mux1/3
  ch-2 voltage/1 -> Mux1/2
  ch-2 power/1 -> Gain1/1
  ch-1 current/1 -> Mux/3
  ch-1 voltage/1 -> Mux/2
  Mux3/1 -> ch [1 2 3]/1

== system NHR9410Model96k_2020b/NHR 9410-96k Input Panel/mode5 ==
  Angle-1 : Constant  Value=0
  Angle-2 : Constant  Value=180
  Angle-3 : Constant  Value=md5ph2
  Frequency-1 : Constant  Value=md5f1
  Frequency-3 : Constant  Value=md5f2
  Gain : Gain  Gain=1000
  Gain1 : Gain  Gain=1000
  Gain2 : Gain  Gain=1000
  Mux{,1..3} (4 alike) : Mux  Inputs=3
  Mux5 : Mux  Inputs=6
  ch-1 current : Constant  Value=md5Irms1
  ch-1 power : Constant  Value=md5Pm1/2
  ch-1 voltage : Constant  Value=md5Vrms1/2
  ch-2 current : Constant  Value=md5Irms1
  ch-2 power : Constant  Value=md5Pm1/2
  ch-2 voltage : Constant  Value=md5Vrms1/2
  ch-3 current : Constant  Value=md5Irms2
  ch-3 power : Constant  Value=md5Pm2
  ch-3 voltage : Constant  Value=md5Vrms2
  ch [1 2 3] : Outport  VectorParamsAs1DForOutWhenUnconnected=off
  F [Angles-1,2,3] : Outport  Port=2  VectorParamsAs1DForOutWhenUnconnected=off
  wires:
  ch-1 voltage/1 -> Mux/2
  Mux3/1 -> ch [1 2 3]/1
  ch-1 current/1 -> Mux/3
  ch-2 power/1 -> Gain1/1
  ch-2 voltage/1 -> Mux1/2
  ch-2 current/1 -> Mux1/3
  ch-3 current/1 -> Mux2/3
  ch-3 voltage/1 -> Mux2/2
  ch-3 power/1 -> Gain2/1
  Mux1/1 -> Mux3/2
  Mux/1 -> Mux3/1
  Mux2/1 -> Mux3/3
  Gain/1 -> Mux/1
  ch-1 power/1 -> Gain/1
  Gain1/1 -> Mux1/1
  Gain2/1 -> Mux2/1
  Angle-1/1 -> Mux5/4
  Frequency-1/1 -> Mux5/2, Mux5/1
  Frequency-3/1 -> Mux5/3
  Angle-2/1 -> Mux5/5
  Angle-3/1 -> Mux5/6
  Mux5/1 -> F [Angles-1,2,3]/1

== system NHR9410Model96k_2020b/NHR 9410-96k Input Panel/mode6 ==
  Angle-1 : Constant  Value=0
  Angle-2 : Constant  Value=180
  Angle-3 : Constant  Value=0
  Frequency-1 : Constant  Value=md6f1
  Frequency-3 : Constant  Value=0
  Gain : Gain  Gain=1000
  Gain1 : Gain  Gain=1000
  Gain2 : Gain  Gain=1000
  Mux{,1..3} (4 alike) : Mux  Inputs=3
  Mux5 : Mux  Inputs=6
  ch-1 current : Constant  Value=md6Irms1
  ch-1 power : Constant  Value=md6Pm1/2
  ch-1 voltage : Constant  Value=md6Vrms1/2
  ch-2 current : Constant  Value=md6Irms1
  ch-2 power : Constant  Value=md6Pm1/2
  ch-2 voltage : Constant  Value=md6Vrms1/2
  ch-3 current : Constant  Value=md6Im2
  ch-3 power : Constant  Value=md6Pm2
  ch-3 voltage : Constant  Value=md6Vm2
  ch [1 2 3] : Outport  VectorParamsAs1DForOutWhenUnconnected=off
  F [Angles-1,2,3] : Outport  Port=2  VectorParamsAs1DForOutWhenUnconnected=off
  wires:
  Gain2/1 -> Mux2/1
  Gain1/1 -> Mux1/1
  ch-1 power/1 -> Gain/1
  Gain/1 -> Mux/1
  Mux2/1 -> Mux3/3
  Mux/1 -> Mux3/1
  Mux1/1 -> Mux3/2
  ch-3 power/1 -> Gain2/1
  ch-3 voltage/1 -> Mux2/2
  ch-3 current/1 -> Mux2/3
  ch-2 current/1 -> Mux1/3
  ch-2 voltage/1 -> Mux1/2
  ch-2 power/1 -> Gain1/1
  ch-1 current/1 -> Mux/3
  Mux3/1 -> ch [1 2 3]/1
  ch-1 voltage/1 -> Mux/2
  Angle-1/1 -> Mux5/4
  Frequency-1/1 -> Mux5/2, Mux5/1
  Frequency-3/1 -> Mux5/3
  Angle-2/1 -> Mux5/5
  Angle-3/1 -> Mux5/6
  Mux5/1 -> F [Angles-1,2,3]/1

== system NHR9410Model96k_2020b/NHR 9410-96k Input Panel/mode7 ==
  Angle-1 : Constant  Value=md7ph1
  Angle-2 : Constant  Value=0
  Angle-3 : Constant  Value=md7ph2
  Frequency-1 : Constant  Value=md7f1
  Frequency-2 : Constant  Value=0
  Frequency-3 : Constant  Value=md7f2
  Gain : Gain  Gain=1000
  Gain1 : Gain  Gain=1000
  Gain2 : Gain  Gain=1000
  Mux{,1..3} (4 alike) : Mux  Inputs=3
  Mux5 : Mux  Inputs=6
  ch-1 current : Constant  Value=md7Irms1
  ch-1 power : Constant  Value=md7Pm1
  ch-1 voltage : Constant  Value=md7Vrms1
  ch-2 current : Constant  Value=0
  ch-2 power : Constant  Value=0
  ch-2 voltage : Constant  Value=0
  ch-3 current : Constant  Value=md7Irms2
  ch-3 power : Constant  Value=md7Pm2
  ch-3 voltage : Constant  Value=md7Vrms2
  ch [1 2 3] : Outport  VectorParamsAs1DForOutWhenUnconnected=off
  F [Angles-1,2,3] : Outport  Port=2  VectorParamsAs1DForOutWhenUnconnected=off
  wires:
  ch-1 voltage/1 -> Mux/2
  Mux3/1 -> ch [1 2 3]/1
  ch-1 current/1 -> Mux/3
  ch-2 power/1 -> Gain1/1
  ch-2 voltage/1 -> Mux1/2
  ch-2 current/1 -> Mux1/3
  ch-3 current/1 -> Mux2/3
  ch-3 voltage/1 -> Mux2/2
  ch-3 power/1 -> Gain2/1
  Mux1/1 -> Mux3/2
  Mux/1 -> Mux3/1
  Mux2/1 -> Mux3/3
  Gain/1 -> Mux/1
  ch-1 power/1 -> Gain/1
  Gain1/1 -> Mux1/1
  Gain2/1 -> Mux2/1
  Angle-1/1 -> Mux5/4
  Frequency-2/1 -> Mux5/2
  Frequency-3/1 -> Mux5/3
  Angle-2/1 -> Mux5/5
  Angle-3/1 -> Mux5/6
  Frequency-1/1 -> Mux5/1
  Mux5/1 -> F [Angles-1,2,3]/1

== system NHR9410Model96k_2020b/NHR 9410-96k Input Panel/mode8 ==
  Angle-1 : Constant  Value=md8ph1
  Angle-2 : Constant  Value=0
  Angle-3 : Constant  Value=0
  Frequency-1 : Constant  Value=md8f1
  Frequency-2 : Constant  Value=0
  Frequency-3 : Constant  Value=0
  Gain : Gain  Gain=1000
  Gain1 : Gain  Gain=1000
  Gain2 : Gain  Gain=1000
  Mux{,1..3} (4 alike) : Mux  Inputs=3
  Mux5 : Mux  Inputs=6
  ch-1 current : Constant  Value=md8Irms1
  ch-1 power : Constant  Value=md8Pm1
  ch-1 voltage : Constant  Value=md8Vrms1
  ch-2 current : Constant  Value=0
  ch-2 power : Constant  Value=0
  ch-2 voltage : Constant  Value=0
  ch-3 current : Constant  Value=md8Im2
  ch-3 power : Constant  Value=md8Pm2
  ch-3 voltage : Constant  Value=md8Vm2
  ch [1 2 3] : Outport  VectorParamsAs1DForOutWhenUnconnected=off
  F [Angles-1,2,3] : Outport  Port=2  VectorParamsAs1DForOutWhenUnconnected=off
  wires:
  Gain2/1 -> Mux2/1
  Gain1/1 -> Mux1/1
  ch-1 power/1 -> Gain/1
  Gain/1 -> Mux/1
  Mux2/1 -> Mux3/3
  Mux/1 -> Mux3/1
  Mux1/1 -> Mux3/2
  ch-3 power/1 -> Gain2/1
  ch-3 voltage/1 -> Mux2/2
  ch-3 current/1 -> Mux2/3
  ch-2 current/1 -> Mux1/3
  ch-2 voltage/1 -> Mux1/2
  ch-2 power/1 -> Gain1/1
  ch-1 current/1 -> Mux/3
  Mux3/1 -> ch [1 2 3]/1
  ch-1 voltage/1 -> Mux/2
  Angle-1/1 -> Mux5/4
  Frequency-2/1 -> Mux5/2
  Frequency-3/1 -> Mux5/3
  Angle-2/1 -> Mux5/5
  Angle-3/1 -> Mux5/6
  Frequency-1/1 -> Mux5/1
  Mux5/1 -> F [Angles-1,2,3]/1

== system NHR9410Model96k_2020b/NHR 9410-96k Input Panel/mode9 ==
  Angle-1 : Constant  Value=md9ph1
  Angle-2 : Constant  Value=md9ph2
  Angle-3 : Constant  Value=0
  Frequency-1 : Constant  Value=md9f1
  Frequency-2 : Constant  Value=md9f2
  Frequency-3 : Constant  Value=0
  Gain : Gain  Gain=1000
  Gain1 : Gain  Gain=1000
  Gain2 : Gain  Gain=1000
  Mux{,1..3} (4 alike) : Mux  Inputs=3
  Mux5 : Mux  Inputs=6
  ch-1 current : Constant  Value=md9Irms1
  ch-1 power : Constant  Value=md9Pm1
  ch-1 voltage : Constant  Value=md9Vrms1
  ch-2 current : Constant  Value=md9Irms2
  ch-2 power : Constant  Value=md9Pm2
  ch-2 voltage : Constant  Value=md9Vrms2
  ch-3 current : Constant  Value=md9Im3
  ch-3 power : Constant  Value=md9Pm3
  ch-3 voltage : Constant  Value=md9Vm3
  ch [1 2 3] : Outport  VectorParamsAs1DForOutWhenUnconnected=off
  F [Angles-1,2,3] : Outport  Port=2  VectorParamsAs1DForOutWhenUnconnected=off
  wires:
  Gain2/1 -> Mux2/1
  Gain1/1 -> Mux1/1
  ch-1 power/1 -> Gain/1
  Gain/1 -> Mux/1
  Mux2/1 -> Mux3/3
  Mux/1 -> Mux3/1
  Mux1/1 -> Mux3/2
  ch-3 power/1 -> Gain2/1
  ch-3 voltage/1 -> Mux2/2
  ch-3 current/1 -> Mux2/3
  ch-2 current/1 -> Mux1/3
  ch-2 voltage/1 -> Mux1/2
  ch-2 power/1 -> Gain1/1
  ch-1 current/1 -> Mux/3
  Mux3/1 -> ch [1 2 3]/1
  ch-1 voltage/1 -> Mux/2
  Angle-1/1 -> Mux5/4
  Frequency-2/1 -> Mux5/2
  Frequency-3/1 -> Mux5/3
  Angle-2/1 -> Mux5/5
  Angle-3/1 -> Mux5/6
  Frequency-1/1 -> Mux5/1
  Mux5/1 -> F [Angles-1,2,3]/1

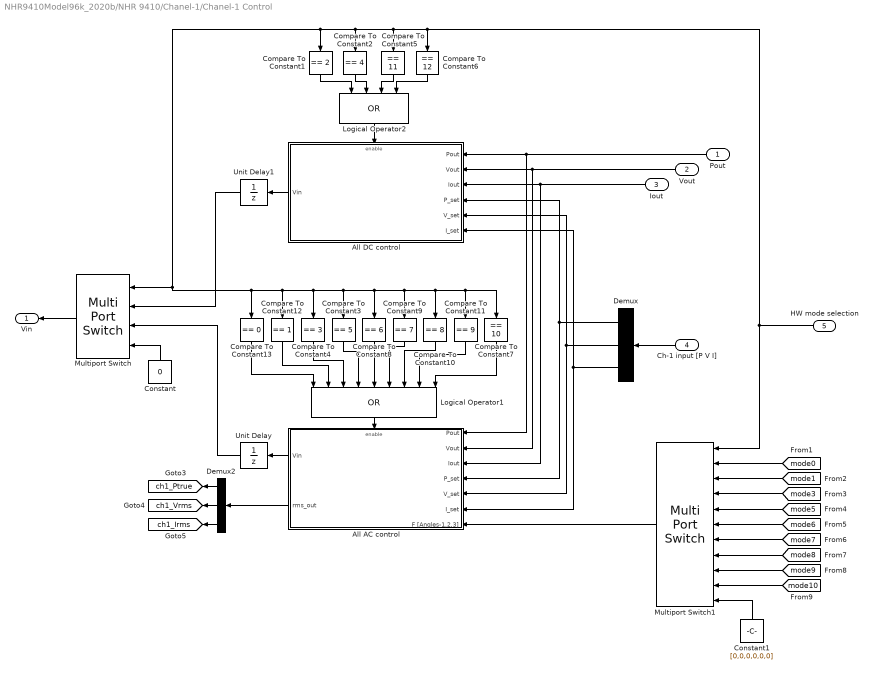
== system NHR9410Model96k_2020b/NHR 9410/Chanel-1/Chanel-1 Control ==
  Pout : Inport
  Vout : Inport  Port=2
  Iout : Inport  Port=3
  Ch-1 input [P V I] : Inport  Port=4
  HW mode selection : Inport  Port=5
  All AC control : Subsystem
      settings: MinAlgLoopOccurrences=on
  All DC control : Subsystem
      settings: MinAlgLoopOccurrences=on
  Compare To Constant1 : simulink/Logic and Bit Operations/Compare To Constant  relop===  const=2  OutDataTypeStr=boolean
  Compare To Constant10 : simulink/Logic and Bit Operations/Compare To Constant  relop===  const=8  OutDataTypeStr=boolean
  Compare To Constant11 : simulink/Logic and Bit Operations/Compare To Constant  relop===  const=9  OutDataTypeStr=boolean
  Compare To Constant12 : simulink/Logic and Bit Operations/Compare To Constant  relop===  const=1  OutDataTypeStr=boolean
  Compare To Constant13 : simulink/Logic and Bit Operations/Compare To Constant  relop===  const=0  OutDataTypeStr=boolean
  Compare To Constant2 : simulink/Logic and Bit Operations/Compare To Constant  relop===  const=4  OutDataTypeStr=boolean
  Compare To Constant3 : simulink/Logic and Bit Operations/Compare To Constant  relop===  const=5  OutDataTypeStr=boolean
  Compare To Constant4 : simulink/Logic and Bit Operations/Compare To Constant  relop===  const=3  OutDataTypeStr=boolean
  Compare To Constant5 : simulink/Logic and Bit Operations/Compare To Constant  relop===  const=11  OutDataTypeStr=boolean
  Compare To Constant6 : simulink/Logic and Bit Operations/Compare To Constant  relop===  const=12  OutDataTypeStr=boolean
  Compare To Constant7 : simulink/Logic and Bit Operations/Compare To Constant  relop===  const=10  OutDataTypeStr=boolean
  Compare To Constant8 : simulink/Logic and Bit Operations/Compare To Constant  relop===  const=6  OutDataTypeStr=boolean
  Compare To Constant9 : simulink/Logic and Bit Operations/Compare To Constant  relop===  const=7  OutDataTypeStr=boolean
  Constant : Constant  Value=0
  Constant1 : Constant  Value=[0,0,0,0,0,0]
  Demux : Demux  Outputs=3
  Demux2 : Demux  Outputs=3
  Logical Operator1 : Logic  Operator=OR  Inputs=9  AllPortsSameDT=off  OutDataTypeStr=boolean
  Logical Operator2 : Logic  Operator=OR  Inputs=4  AllPortsSameDT=off  OutDataTypeStr=boolean
  Multiport Switch : MultiPortSwitch  DataPortOrder=Specify indices  Inputs=13  DataPortIndices={[2,4,11,12],[0,1,3,5,6,7,8,9,10]}  DataPortForDefault=Additional data port  DiagnosticForDefault=None
  Multiport Switch1 : MultiPortSwitch  DataPortOrder=Specify indices  Inputs=13  DataPortIndices={0,1,3,5,6,7,8,9,10}  DataPortForDefault=Additional data port  DiagnosticForDefault=None
  Unit Delay : UnitDelay  SampleTime=-1  HasFrameUpgradeWarning=on
  Unit Delay1 : UnitDelay  SampleTime=-1  HasFrameUpgradeWarning=on
  Vin : Outport  VectorParamsAs1DForOutWhenUnconnected=off
  tag scope: ch1_Irms=global, ch1_Ptrue=global, ch1_Vrms=global
  wires:
  Compare To Constant2/1 -> Logical Operator2/2
  Compare To Constant1/1 -> Logical Operator2/1
  HW mode selection/1 -> Multiport Switch1/1, Compare To Constant6/1, Compare To Constant5/1, Compare To Constant2/1, Compare To Constant1/1, Multiport Switch/1, Compare To Constant13/1, Compare To Constant12/1, Compare To Constant3/1, Compare To Constant7/1, Compare To Constant11/1, Compare To Constant10/1, Compare To Constant9/1, Compare To Constant8/1, Compare To Constant4/1
  All AC control/1(Vin) -> Unit Delay/1
  All DC control/1(Vin) -> Unit Delay1/1
  All AC control/2(rms_out) -> Demux2/1
  Logical Operator1/1 -> All AC control/Enable
  Logical Operator2/1 -> All DC control/Enable
  Constant/1 -> Multiport Switch/4
  Multiport Switch/1 -> Vin/1
  Pout/1 -> All DC control/1(Pout), All AC control/1(Pout)
  Iout/1 -> All DC control/3(Iout), All AC control/3(Iout)
  Demux2/1 -> [ch1_Ptrue]
  Demux2/3 -> [ch1_Irms]
  Demux2/2 -> [ch1_Vrms]
  Vout/1 -> All DC control/2(Vout), All AC control/2(Vout)
  Ch-1 input [P V I]/1 -> Demux/1
  Demux/1 -> All AC control/4(P_set), All DC control/4(P_set)
  Demux/2 -> All AC control/5(V_set), All DC control/5(V_set)
  Demux/3 -> All AC control/6(I_set), All DC control/6(I_set)
  Compare To Constant5/1 -> Logical Operator2/3
  Compare To Constant6/1 -> Logical Operator2/4
  Compare To Constant8/1 -> Logical Operator1/5
  Compare To Constant9/1 -> Logical Operator1/6
  Compare To Constant10/1 -> Logical Operator1/7
  Compare To Constant11/1 -> Logical Operator1/8
  Compare To Constant7/1 -> Logical Operator1/9
  Compare To Constant13/1 -> Logical Operator1/1
  Compare To Constant12/1 -> Logical Operator1/2
  Compare To Constant4/1 -> Logical Operator1/3
  Compare To Constant3/1 -> Logical Operator1/4
  [mode0] -> Multiport Switch1/2
  [mode1] -> Multiport Switch1/3
  [mode3] -> Multiport Switch1/4
  [mode5] -> Multiport Switch1/5
  [mode6] -> Multiport Switch1/6
  [mode7] -> Multiport Switch1/7
  [mode8] -> Multiport Switch1/8
  [mode9] -> Multiport Switch1/9
  [mode10] -> Multiport Switch1/10
  Constant1/1 -> Multiport Switch1/11
  Multiport Switch1/1 -> All AC control/7(F [Angles-1,2,3])
  Unit Delay/1 -> Multiport Switch/3
  Unit Delay1/1 -> Multiport Switch/2

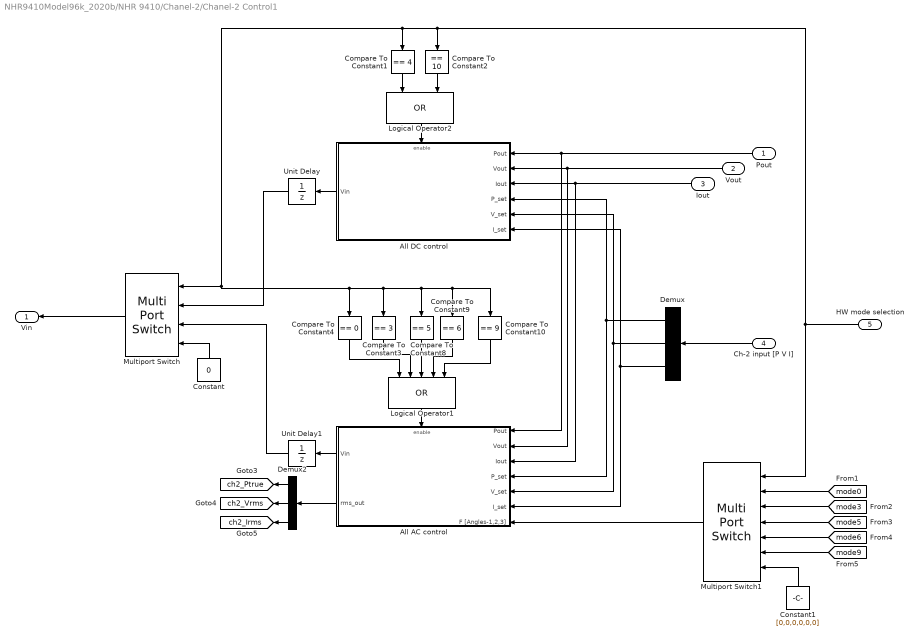
== system NHR9410Model96k_2020b/NHR 9410/Chanel-2/Chanel-2 Control1 ==
  Pout : Inport
  Vout : Inport  Port=2
  Iout : Inport  Port=3
  Ch-2 input [P V I] : Inport  Port=4
  HW mode selection : Inport  Port=5
  All AC control : Subsystem
      settings: MinAlgLoopOccurrences=on
  All DC control : Subsystem
      settings: MinAlgLoopOccurrences=on
  Compare To Constant1 : simulink/Logic and Bit Operations/Compare To Constant  relop===  const=4  OutDataTypeStr=boolean
  Compare To Constant10 : simulink/Logic and Bit Operations/Compare To Constant  relop===  const=9  OutDataTypeStr=boolean
  Compare To Constant2 : simulink/Logic and Bit Operations/Compare To Constant  relop===  const=10  OutDataTypeStr=boolean
  Compare To Constant3 : simulink/Logic and Bit Operations/Compare To Constant  relop===  const=3  OutDataTypeStr=boolean
  Compare To Constant4 : simulink/Logic and Bit Operations/Compare To Constant  relop===  const=0  OutDataTypeStr=boolean
  Compare To Constant8 : simulink/Logic and Bit Operations/Compare To Constant  relop===  const=5  OutDataTypeStr=boolean
  Compare To Constant9 : simulink/Logic and Bit Operations/Compare To Constant  relop===  const=6  OutDataTypeStr=boolean
  Constant : Constant  Value=0
  Constant1 : Constant  Value=[0,0,0,0,0,0]
  Demux : Demux  Outputs=3
  Demux2 : Demux  Outputs=3
  Logical Operator1 : Logic  Operator=OR  Inputs=5  AllPortsSameDT=off  OutDataTypeStr=boolean
  Logical Operator2 : Logic  Operator=OR  AllPortsSameDT=off  OutDataTypeStr=boolean
  Multiport Switch : MultiPortSwitch  DataPortOrder=Specify indices  Inputs=13  DataPortIndices={[4,10],[0,3,5,6,9]}  DataPortForDefault=Additional data port  DiagnosticForDefault=None
  Multiport Switch1 : MultiPortSwitch  DataPortOrder=Specify indices  Inputs=13  DataPortIndices={0,3,5,6,9}  DataPortForDefault=Additional data port  DiagnosticForDefault=None
  Unit Delay : UnitDelay  SampleTime=-1  HasFrameUpgradeWarning=on
  Unit Delay1 : UnitDelay  SampleTime=-1  HasFrameUpgradeWarning=on
  Vin : Outport  VectorParamsAs1DForOutWhenUnconnected=off
  tag scope: ch2_Irms=global, ch2_Ptrue=global, ch2_Vrms=global
  wires:
  Demux/3 -> All DC control/6(I_set), All AC control/6(I_set)
  Demux/2 -> All DC control/5(V_set), All AC control/5(V_set)
  Demux/1 -> All DC control/4(P_set), All AC control/4(P_set)
  Ch-2 input [P V I]/1 -> Demux/1
  Vout/1 -> All DC control/2(Vout), All AC control/2(Vout)
  Demux2/2 -> [ch2_Vrms]
  Demux2/3 -> [ch2_Irms]
  Demux2/1 -> [ch2_Ptrue]
  Iout/1 -> All DC control/3(Iout), All AC control/3(Iout)
  Pout/1 -> All DC control/1(Pout), All AC control/1(Pout)
  Multiport Switch/1 -> Vin/1
  Constant/1 -> Multiport Switch/4
  Logical Operator2/1 -> All DC control/Enable
  Compare To Constant4/1 -> Logical Operator1/1
  Compare To Constant3/1 -> Logical Operator1/2
  Compare To Constant8/1 -> Logical Operator1/3
  Compare To Constant9/1 -> Logical Operator1/4
  Compare To Constant10/1 -> Logical Operator1/5
  Logical Operator1/1 -> All AC control/Enable
  All AC control/2(rms_out) -> Demux2/1
  All DC control/1(Vin) -> Unit Delay/1
  All AC control/1(Vin) -> Unit Delay1/1
  Multiport Switch1/1 -> All AC control/7(F [Angles-1,2,3])
  HW mode selection/1 -> Compare To Constant4/1, Compare To Constant10/1, Compare To Constant9/1, Compare To Constant8/1, Compare To Constant3/1, Multiport Switch/1, Compare To Constant1/1, Compare To Constant2/1, Multiport Switch1/1
  [mode0] -> Multiport Switch1/2
  [mode3] -> Multiport Switch1/3
  [mode5] -> Multiport Switch1/4
  [mode6] -> Multiport Switch1/5
  [mode9] -> Multiport Switch1/6
  Constant1/1 -> Multiport Switch1/7
  Compare To Constant1/1 -> Logical Operator2/1
  Compare To Constant2/1 -> Logical Operator2/2
  Unit Delay/1 -> Multiport Switch/2
  Unit Delay1/1 -> Multiport Switch/3
